simulink model "simple_led_task"  (Simulink 3.00)
libraries: logiclib x7, mathlib x5, execlib x2, inoutlib x1

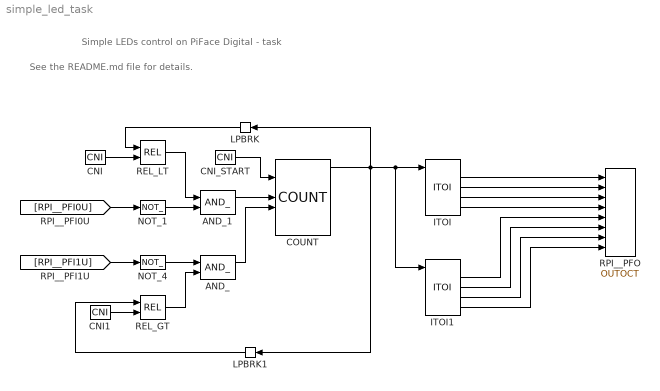
== system simple_led_task ==
  note: See the README.md file for details.
  note: Simple LEDs control on PiFace Digital - task
  AND_ : logiclib/AND_
  AND_1 : logiclib/AND_
  CNI : mathlib/CNI  icn=8
  CNI1 : mathlib/CNI  icn=0
  CNI_START : mathlib/CNI  icn=3
  COUNT : logiclib/COUNT
  ITOI : logiclib/ITOI  BINF=off  fktab=[0 1 2 4 8 0 0 0 0 0 0 0 0 0 0 0]
  ITOI1 : logiclib/ITOI  BINF=off  fktab=[0 0 0 0 0 1 2 4 8 0 0 0 0 0 0 0]
  LPBRK : execlib/LPBRK  Orientation=left
  LPBRK1 : execlib/LPBRK  Orientation=left
  NOT_1 : logiclib/NOT_
  NOT_4 : logiclib/NOT_
  REL_GT : mathlib/REL  irel=4: greater than (>)
  REL_LT : mathlib/REL  irel=3: less than (<)
  RPI__PFO : inoutlib/OUTOCT
  wires:
  AND_/1 -> COUNT/5
  AND_1/1 -> COUNT/4
  CNI/1 -> REL_LT/2
  CNI1/1 -> REL_GT/2
  CNI_START/1 -> COUNT/2
  COUNT/1 -> ITOI/1, ITOI1/1, LPBRK/1, LPBRK1/1
  ITOI/2 -> RPI__PFO/1
  ITOI/3 -> RPI__PFO/2
  ITOI/4 -> RPI__PFO/3
  ITOI/5 -> RPI__PFO/4
  ITOI1/2 -> RPI__PFO/5
  ITOI1/3 -> RPI__PFO/6
  ITOI1/4 -> RPI__PFO/7
  ITOI1/5 -> RPI__PFO/8
  LPBRK/1 -> REL_LT/1
  LPBRK1/1 -> REL_GT/1
  NOT_1/1 -> AND_1/2
  NOT_4/1 -> AND_/1
  REL_GT/1 -> AND_/2
  REL_LT/1 -> AND_1/1
  [RPI__PFI0U] -> NOT_1/1
  [RPI__PFI1U] -> NOT_4/1
